simulink subsystem "Simulation"  (R2025b)
settings: Solver=VariableStepAuto  StartTime=0.0  StopTime=10.0  RelTol=1e-3
undefined symbols (not defined in the file or in its folder): angular_velocity, AUV, data, data_SL_Info, elevation, fractalcoef, heading, height, linear_acceleration, orientation, Sim3dSensor, Simple, T200, thruster_pose, width, x_vel_btm, XYZ, y_vel_btm, z_vel_btm
libraries: ros2lib x15, sim3dlib x7, robotcorelib x5, AUVLib x4, aerolib6dof2 x2, sim3dcameralib x2, matrix_library x1, mspsensorlib x1, aerolibutil x1, mspfiltlib x1
(part 2 of 2)

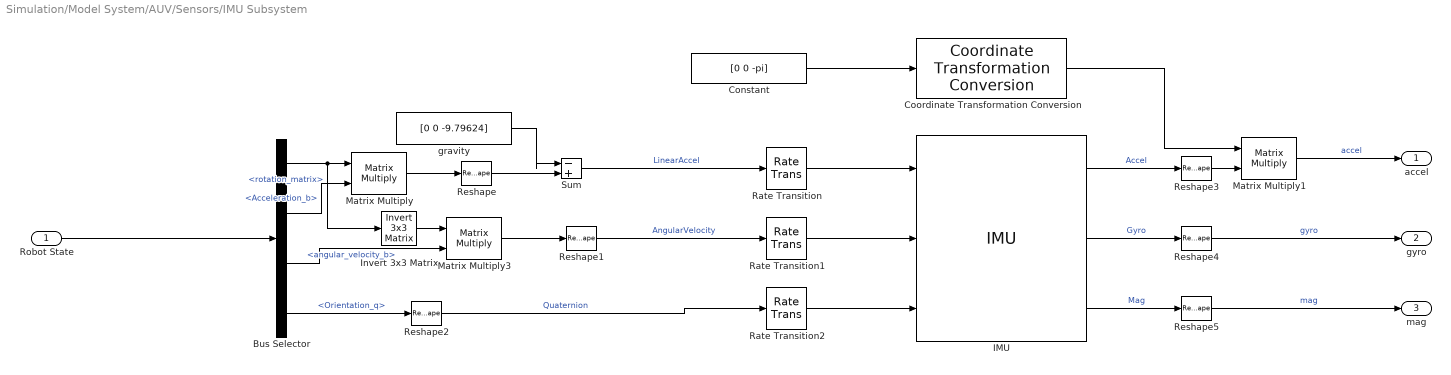
== system Simulation/Model System/AUV/Sensors/IMU Subsystem ==
  Robot State : Inport
  Bus Selector : BusSelector  OutputSignals=rotation_matrix,Acceleration_b,angular_velocity_b,Orientation_q
  Constant : Constant  Value=[0 0 -pi]
  Coordinate Transformation Conversion : robotcorelib/Coordinate Transformation Conversion  InputRepresentation=Euler Angles  InputEulerSequence=ZYX  ShowTrVecInputPort=on  OutputRepresentation=Rotation Matrix  OutputEulerSequence=ZYX  ShowTrVecOutputPort=on  SimulateUsing=Interpreted execution
      settings: LibrarySourceBlock=navlib/Utilities/Coordinate Transformation Conversion
  IMU : mspsensorlib/IMU  DispRefFrame=NED  TemperaturePort=off  Temperature=Temperature  MagneticFieldPort=off  MagneticFieldNED=MagneticFieldNED  MagneticFieldENU=[ -2.4169, 27.5550, 16.0849 ]  SeedDouble=67  SimulateUsing=Interpreted execution  AccelParamsMeasurementRange=AccelParamsMeasurementRange  AccelParamsResolution=AccelParamsResolution  AccelParamsConstantBias=AccelParamsConstantBias  AccelParamsAxesMisalignment=AccelParamsAxesMisalignment  AccelParamsNoiseDensity=AccelParamsNoiseDensity  AccelParamsBiasInstability=AccelParamsBiasInstability  AccelParamsBiasInstabilityNumerator=AccelParamsBiasInstabilityNumerator  AccelParamsBiasInstabilityDenominator=AccelParamsBiasInstabilityDenominator  AccelParamsRandomWalk=AccelParamsRandomWalk  AccelParamsNoiseType=double-sided  AccelParamsTemperatureBias=AccelParamsTemperatureBias  AccelParamsTemperatureScaleFactor=AccelParamsTemperatureScaleFactor  GyroParamsMeasurementRange=GyroParamsMeasurementRange  GyroParamsResolution=GyroParamsResolution  GyroParamsConstantBias=GyroParamsConstantBias  GyroParamsAxesMisalignment=GyroParamsAxesMisalignment  GyroParamsAccelerationBias=GyroParamsAccelerationBias  GyroParamsNoiseDensity=GyroParamsNoiseDensity  GyroParamsBiasInstability=GyroParamsBiasInstability  GyroParamsBiasInstabilityNumerator=GyroParamsBiasInstabilityNumerator  GyroParamsBiasInstabilityDenominator=GyroParamsBiasInstabilityDenominator  GyroParamsRandomWalk=GyroParamsRandomWalk  GyroParamsNoiseType=double-sided  GyroParamsTemperatureBias=GyroParamsTemperatureBias  GyroParamsTemperatureScaleFactor=GyroParamsTemperatureScaleFactor  MagParamsMeasurementRange=MagParamsMeasurementRange  MagParamsResolution=MagParamsResolution  MagParamsConstantBias=MagParamsConstantBias  MagParamsAxesMisalignment=MagParamsAxesMisalignment  MagParamsNoiseDensity=MagParamsNoiseDensity  MagParamsBiasInstability=MagParamsBiasInstability  MagParamsBiasInstabilityNumerator=MagParamsBiasInstabilityNumerator  MagParamsBiasInstabilityDenominator=MagParamsBiasInstabilityDenominator  MagParamsRandomWalk=MagParamsRandomWalk  MagParamsNoiseType=double-sided  MagParamsTemperatureBias=MagParamsTemperatureBias  MagParamsTemperatureScaleFactor=MagParamsTemperatureScaleFactor
  Invert 3x3 Matrix : aerolibutil/Invert  3x3 Matrix
  Matrix Multiply : Product  Multiplication=Matrix(*)
  Matrix Multiply1 : Product  Multiplication=Matrix(*)
  Matrix Multiply3 : Product  Multiplication=Matrix(*)
  Rate Transition : RateTransition
  Rate Transition1 : RateTransition
  Rate Transition2 : RateTransition
  Reshape : Reshape  OutputDimensionality=Row vector (2-D)
  Reshape1 : Reshape  OutputDimensionality=Row vector (2-D)
  Reshape2 : Reshape  OutputDimensionality=Row vector (2-D)
  Reshape3 : Reshape  OutputDimensionality=Column vector (2-D)
  Reshape4 : Reshape  OutputDimensionality=Column vector (2-D)
  Reshape5 : Reshape  OutputDimensionality=Column vector (2-D)
  Sum : Sum  Inputs=|-+
  gravity : Constant  Value=[0 0 -9.79624]
  accel : Outport
  gyro : Outport  Port=2
  mag : Outport  Port=3
  wires:
  Reshape2/1 -> Rate Transition2/1  "Quaternion"
  Reshape5/1 -> mag/1  "mag"
  Reshape4/1 -> gyro/1  "gyro"
  IMU/3 -> Reshape5/1  "Mag"
  Reshape1/1 -> Rate Transition1/1  "AngularVelocity"
  Reshape3/1 -> Matrix Multiply1/2
  Bus Selector/1 -> Matrix Multiply/1, Invert 3x3 Matrix/1  "<rotation_matrix>"
  Constant/1 -> Coordinate Transformation Conversion/1
  Robot State/1 -> Bus Selector/1
  IMU/1 -> Reshape3/1  "Accel"
  Bus Selector/4 -> Reshape2/1  "<Orientation_q>"
  Bus Selector/2 -> Matrix Multiply/2  "<Acceleration_b>"
  Coordinate Transformation Conversion/1 -> Matrix Multiply1/1
  Rate Transition/1 -> IMU/1
  Matrix Multiply3/1 -> Reshape1/1
  Matrix Multiply/1 -> Reshape/1
  IMU/2 -> Reshape4/1  "Gyro"
  Matrix Multiply1/1 -> accel/1  "accel"
  Invert 3x3 Matrix/1 -> Matrix Multiply3/1
  Sum/1 -> Rate Transition/1  "LinearAccel"
  Bus Selector/3 -> Matrix Multiply3/2  "<angular_velocity_b>"
  Reshape/1 -> Sum/2
  gravity/1 -> Sum/1
  Rate Transition2/1 -> IMU/3
  Rate Transition1/1 -> IMU/2

== system Simulation/Model System/AUV/AUV Dynamics/Thruster Forces and Moments/For Each Subsystem ==
  thruster pose : Inport  Partition=on  PartitionDimension=1  PartitionWidth=1  PartitionOffset=0
  thrust : Inport  Port=2  Partition=on  PartitionDimension=1  PartitionWidth=1  PartitionOffset=0
  Calculate Force and Moment : Subsystem
  For Each : ForEach  DisableCoverage=on
  force : Outport  ConcatenationDimension=1
  moment : Outport  Port=2  ConcatenationDimension=1
  wires:
  thrust/1 -> Calculate Force and Moment/2(Thrust)
  Calculate Force and Moment/1(force) -> force/1
  Calculate Force and Moment/2(moment) -> moment/1
  thruster pose/1 -> Calculate Force and Moment/1(thruster pose)

== system Simulation/Model System/AUV/Actuators/Marker/Marker Dynamics ==
  Initial_state : Inport
  drop_marker : EnablePort
  Bus Selector : BusSelector  OutputSignals=Position_e,Veloctiy_e,rotation_matrix
  Constant : Constant  Value=[marker_pos(1) marker_pos(2) -marker_pos(3)]
  MATLAB Function : MATLAB Function  TreatAsAtomicUnit=on
  Scope : Scope
      settings: ActiveDisplayYMinimum=-8.92103223977475  ActiveDisplayYMaximum=3.8325960679282667  DataLoggingVariableName=ScopeData4
  marker_position : Outport
  wires:
  Constant/1 -> MATLAB Function/4(marker_loc_b)
  Bus Selector/3 -> MATLAB Function/3(rot_m)  "<rotation_matrix>"
  Bus Selector/2 -> MATLAB Function/2(init_velocity)  "<Veloctiy_e>"
  Bus Selector/1 -> MATLAB Function/1(init_pos)  "<Position_e>"
  Initial_state/1 -> Bus Selector/1
  MATLAB Function/1(marker_position) -> marker_position/1, Scope/1

== system Simulation/Model System/AUV/Actuators/Tropedo/Torpedo Dynamics ==
  Initial_state : Inport
  Launch_torpedo : EnablePort
  6DOF (Quaternion) : EOM6DOFBodyQuat  xme_0=torp_pos  Vm_0=[10 0 0]  mass_0=0.02  inertia=[0.02 0 0; 0 0.5 0; 0 0 0.5]
  Bus Creator : BusCreator  Inputs=4
  Bus Creator1 : BusCreator  Inputs=2
  Constant1 : Constant  Value=eye(3)
  Coordinate Transformation Conversion4 : robotcorelib/Coordinate Transformation Conversion  InputRepresentation=Rotation Matrix  InputEulerSequence=ZYX  ShowTrVecInputPort=on  OutputRepresentation=Euler Angles  OutputEulerSequence=XYZ  ShowTrVecOutputPort=on  SimulateUsing=Interpreted execution
      settings: LibrarySourceBlock=navlib/Utilities/Coordinate Transformation Conversion
  Divide1 : Product  Inputs=*/  Multiplication=Matrix(*)
  Environmental Forces and Moments : AUVLib/Environmental Forces and Moments  V=4.041e-5  h=0.01  mass=0.02  CoB=[0; 0; 0]  Hy=Simple  ang_coeff="diag([ 0.3,  2,  20])"  quad_coeff="diag([ 0.05,  1.5,  1.6])"  lin_coeff="diag([ 0.05,  1.5,  1.5])"  ang_coeff_c="diag([ 10, 80,  82])"  alphaR=0  betaR=0  CX=0  CY=0  CZ=0  CMK=0  CMM=0  CMN=0  inputAxes=Body  cbar=1  b=1  S=1
  Subsystem1 : Subsystem
  Torpedo Pose : Outport
  wires:
  Divide1/1 -> Coordinate Transformation Conversion4/1  "rotation_matrix"
  Constant1/1 -> Divide1/1
  Subsystem1/2(rotation_matrix) -> Bus Creator/2, Divide1/2
  Subsystem1/1(Position_e) -> Bus Creator1/2, Bus Creator/1
  6DOF (Quaternion)/6 -> Bus Creator/3  "Velocity_b"
  6DOF (Quaternion)/7 -> Bus Creator/4  "angular_velocity_b"
  6DOF (Quaternion)/5 -> Subsystem1/3(rot_m)  "rotation_matrix"
  6DOF (Quaternion)/2 -> Subsystem1/2(pos_e)  "Position_e"
  Environmental Forces and Moments/2 -> 6DOF (Quaternion)/2
  Environmental Forces and Moments/1 -> 6DOF (Quaternion)/1
  Bus Creator1/1 -> Torpedo Pose/1
  Coordinate Transformation Conversion4/1 -> Bus Creator1/1  "orientation_topedo"
  Initial_state/1 -> Subsystem1/1(init_state)
  Bus Creator/1 -> Environmental Forces and Moments/1  "tropedo_state"

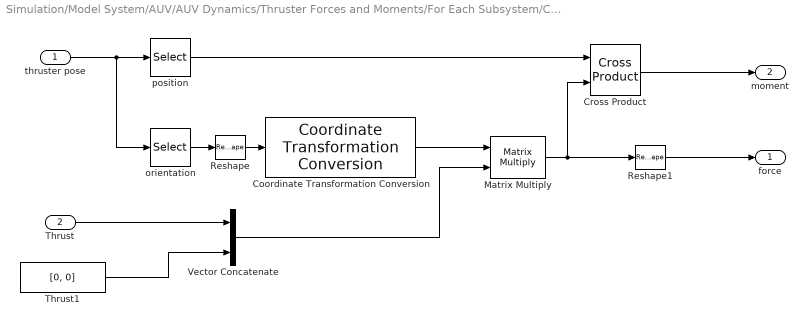
== system Simulation/Model System/AUV/AUV Dynamics/Thruster Forces and Moments/For Each Subsystem/Calculate Force and Moment ==
  thruster pose : Inport
  Thrust : Inport  Port=2
  Coordinate Transformation Conversion : robotcorelib/Coordinate Transformation Conversion  InputRepresentation=Euler Angles  InputEulerSequence=XYZ  ShowTrVecInputPort=on  OutputRepresentation=Rotation Matrix  OutputEulerSequence=ZYX  ShowTrVecOutputPort=on  SimulateUsing=Interpreted execution
  Cross Product : matrix_library/Cross Product
  Matrix Multiply : Product  Multiplication=Matrix(*)
  Reshape : Reshape  OutputDimensionality=Column vector (2-D)
  Reshape1 : Reshape  OutputDimensionality=Row vector (2-D)
  Thrust1 : Constant  Value=[0, 0]
  Vector Concatenate : Concatenate
  orientation : Selector  InputPortWidth=6  IndexOptions=Index vector (dialog)  Indices=[4 5 6]  OutputSizes=1
  position : Selector  InputPortWidth=6  IndexOptions=Index vector (dialog)  Indices=[1 2 3]  OutputSizes=1
  force : Outport
  moment : Outport  Port=2
  wires:
  Reshape1/1 -> force/1
  Reshape/1 -> Coordinate Transformation Conversion/1
  position/1 -> Cross Product/1
  thruster pose/1 -> position/1, orientation/1
  Cross Product/1 -> moment/1
  Thrust/1 -> Vector Concatenate/1
  orientation/1 -> Reshape/1
  Coordinate Transformation Conversion/1 -> Matrix Multiply/1
  Matrix Multiply/1 -> Cross Product/2, Reshape1/1
  Thrust1/1 -> Vector Concatenate/2
  Vector Concatenate/1 -> Matrix Multiply/2

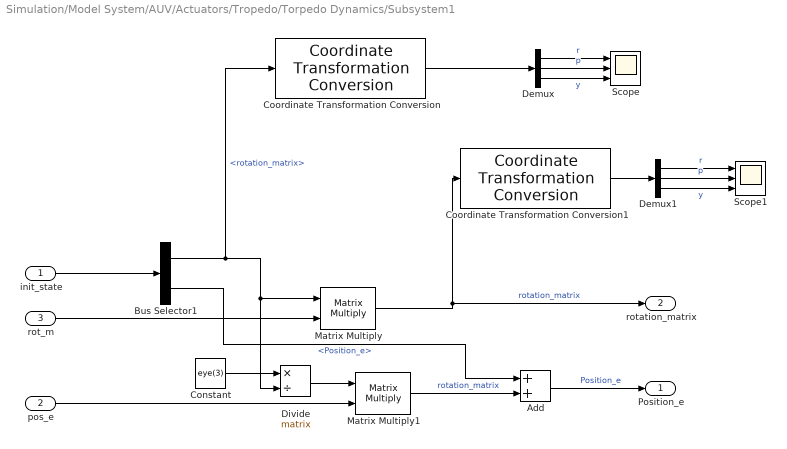
== system Simulation/Model System/AUV/Actuators/Tropedo/Torpedo Dynamics/Subsystem1 ==
  init_state : Inport
  pos_e : Inport  Port=2
  rot_m : Inport  Port=3
  Add : Sum
  Bus Selector1 : BusSelector  OutputSignals=rotation_matrix,Position_e
  Constant : Constant  Value=eye(3)
  Coordinate Transformation Conversion : robotcorelib/Coordinate Transformation Conversion  InputRepresentation=Rotation Matrix  InputEulerSequence=ZYX  ShowTrVecInputPort=on  OutputRepresentation=Euler Angles  OutputEulerSequence=XYZ  ShowTrVecOutputPort=on  SimulateUsing=Interpreted execution
      settings: LibrarySourceBlock=navlib/Utilities/Coordinate Transformation Conversion
  Coordinate Transformation Conversion1 : robotcorelib/Coordinate Transformation Conversion  InputRepresentation=Rotation Matrix  InputEulerSequence=ZYX  ShowTrVecInputPort=on  OutputRepresentation=Euler Angles  OutputEulerSequence=XYZ  ShowTrVecOutputPort=on  SimulateUsing=Interpreted execution
      settings: LibrarySourceBlock=navlib/Utilities/Coordinate Transformation Conversion
  Demux : Demux  Outputs=3
  Demux1 : Demux  Outputs=3
  Divide : Product  Inputs=*/  Multiplication=Matrix(*)
  Matrix Multiply : Product  Multiplication=Matrix(*)
  Matrix Multiply1 : Product  Multiplication=Matrix(*)
  Scope : Scope  NumInputPorts=3
      settings: ActiveDisplayYMinimum=-0.91505450914068209  ActiveDisplayYMaximum=0.11578058031846855  DataLoggingVariableName=ScopeData12
  Scope1 : Scope  NumInputPorts=3
      settings: ActiveDisplayYMinimum=-0.098174770424681021  ActiveDisplayYMaximum=0.88357293382212942  DataLoggingVariableName=ScopeData13
  Position_e : Outport
  rotation_matrix : Outport  Port=2
  wires:
  Matrix Multiply/1 -> rotation_matrix/1, Coordinate Transformation Conversion1/1  "rotation_matrix"
  Demux1/3 -> Scope1/3  "y"
  Demux1/2 -> Scope1/2  "p"
  Demux1/1 -> Scope1/1  "r"
  Demux/3 -> Scope/3  "y"
  Demux/1 -> Scope/1  "r"
  Demux/2 -> Scope/2  "p"
  Coordinate Transformation Conversion1/1 -> Demux1/1
  Coordinate Transformation Conversion/1 -> Demux/1
  Add/1 -> Position_e/1  "Position_e"
  Matrix Multiply1/1 -> Add/2  "rotation_matrix"
  Divide/1 -> Matrix Multiply1/1
  Constant/1 -> Divide/1
  pos_e/1 -> Matrix Multiply1/2
  rot_m/1 -> Matrix Multiply/2
  init_state/1 -> Bus Selector1/1
  Bus Selector1/2 -> Add/1  "<Position_e>"
  Bus Selector1/1 -> Matrix Multiply/1, Divide/2, Coordinate Transformation Conversion/1  "<rotation_matrix>"

== matlab function Simulation/ROS Output/Send Depth msg1/MATLAB Function ==
  data: image input; H output; W output; Data output; DataLength output
function [H,W,Data,DataLength] = fcn(image)
[H,W,n]=size(image);

image= permute(image,[3 2 1]);
Data = image(:);
DataLength=uint32(H*W*n);

== matlab function Simulation/ROS Output/Send Depth msg1/MATLAB Function1 ==
  data: image input; H output; W output; Data output; DataLength output
function [H,W,Data,DataLength] = fcn(image)
[H,W,n]=size(image);
H = uint32(H);
W= uint32(W);

Data = image(:);
DataLength=uint32(H*W*n);

== matlab function Simulation/ROS Output/Send Depth msg1/MATLAB Function2 ==
  data: image input; H output; W output; Data output; DataLength output
function [H,W,Data,DataLength] = fcn(image)
[H,W,n]=size(image);
image= permute(image,[3 2 1]);
Data = image(:);

DataLength=uint32(H*W*n);

== matlab function Simulation/Model System/AUV/Actuators/Marker/Marker Dynamics/MATLAB Function ==
  data: init_pos input; init_velocity input; marker_position output; rot_m input; marker_loc_b input
function marker_position = marker_traj(init_pos, init_velocity, rot_m, marker_loc_b)

%Get initial position in inertial frame
position_0 = (eye(3)\rot_m)*marker_loc_b + init_pos;

g = 9.79624;
a = [0 0 g]';

persistent position_t
if isempty(position_t)
    position_t = position_0;
end

persistent velocity
if isempty(velocity)
    velocity = init_velocity;
end

%sample time
dt = 0.01;

% Update position using Newton's equations of motion
% position_t(1) = position_t(1) + velocity(1)*dt;
% position_t(2) = position_t(2) + velocity(2)*dt;
% position_t(3) = position_t(3) + velocity(3)*dt + 0.5*g*dt^2;
position_t = position_t + velocity.*dt + 0.5.*a.*dt^2;

% Velocity updated with uniform drag in all axes (assuming a sphere)
velocity = velocity + a.*dt - (diag([0.02 0.02 0.02]) * velocity);

% set z position to pool floor once it reaches/exceeds pool depth
if position_t(3) > 0.4
    position_t(3) = 0.4;
end

marker_position = position_t;

== matlab function Simulation/Model System/AUV/Sensors/DVL ==
  settings: updateMethod=DISCRETE
  data: body_vel input; vel_b_dvl output; position_e input; rot_m input; v_current_e input; reference_mode input; altitude_dvl output; vel_cov_diag_dvl output; reference output
function [vel_b_dvl, altitude_dvl, vel_cov_diag_dvl, reference] = dvl_sim(body_vel, position_e, rot_m, v_current_e, reference_mode)

seafloor_depth = 2.25; %Depth of pool in m
depth = position_e(3) + 2.2;

vel_b_dvl = zeros([3,1]);

% Noise (1-sigma) in m/s; typical small DVL ~ 0.003–0.02 m/s
% sigma_xyz = [0.01; 0.01; 0.015];
sigma_xyz = [0; 0; 0];

% Slow bias as Gauss-Markov (per axis)
tau_bias = 300.0;         % s, time constant of bias drift (5 min)
sigma_bias_ss = 0.01;     % m/s, steady-state std dev of bias
dt = 0.01;                % s, assumed sample time for bias update


persistent bxyz
if isempty(bxyz)
    bxyz = zeros(3,1);
end

v_b_true = body_vel;

reference = uint8(reference_mode);
if reference == uint8(1) % bottom-track
    v_rel_b = v_b_true;
elseif reference == uint8(2) % water-track
    v_rel_b = v_b_true + (rot_m * v_current_e);
else
    % Unknown: default to bottom-track behavior
    v_rel_b = v_b_true;
    reference = uint8(0);
end

if ~isnan(depth) && ~isnan(seafloor_depth)
    altitude_dvl = max(seafloor_depth - depth, 0.0);
else
    altitude_dvl = NaN;
end

% ---------------- Update bias (Gauss-Markov) ----------------
if tau_bias > 0 && sigma_bias_ss > 0
    % Discrete-time OU: b_{k+1} = (1 - dt/tau) b_k + sqrt(2*sigma^2*dt/tau) * w
    a = max(0.0, 1.0 - dt/tau_bias);
    q = sqrt(max(0.0, 2.0*sigma_bias_ss^2*dt/tau_bias));
    bxyz = a*bxyz + q * randn(3,1);
else
    bxyz = zeros(3,1);
end

% ---------------- Add noise & bias ----------------
eps_xyz = sigma_xyz .* randn(3,1);    % white noise
vel_b_dvl = v_rel_b + bxyz + eps_xyz;

vel_cov_diag_dvl = sigma_xyz.^2;
